simulink model "ARC_DTm"  (R2025b)
settings: Solver=FixedStepAuto  StartTime=0.0  StopTime=10080  FixedStep=1  RelTol=1e-3
PreLoadFcn:
  | %For Preload, set the working path
  | modelFolder = fileparts(which(bdroot));
  | addpath(genpath(modelFolder));
StartFcn:
  | tic
StopFcn:
  | fprintf("Sim Time: %.02f min", toc/60)
values from neighbouring files (symbols this model uses):
  batteryScenario = p.batteryScenario    [RUNSIM_ParameterSweep.m]    (also in _RUNSIM_ParameterSweep.m)
  Electricity_SalePriceModifier = 50/100    (= 0.5)    [RUNSIM_ParameterSweep.m]    (also in _RUNSIM_ParameterSweep.m)
  LUT = LUT_load.gamLUT    [RUNSIM_ParameterSweep.m]    (also in _RUNSIM_ParameterSweep.m)
  minimum_UF_system_flow = 5833    [RUNSIM_ParameterSweep.m]    (also in _RUNSIM_ParameterSweep.m)
  PROS1_recoveryrate = 61    [RUNSIM_ParameterSweep.m]    (also in _RUNSIM_ParameterSweep.m)
  PROS2_recoveryrate = 62    [RUNSIM_ParameterSweep.m]    (also in _RUNSIM_ParameterSweep.m)
  ROstabilization_time = p.ROstabilization_time    [RUNSIM_ParameterSweep.m]    (also in _RUNSIM_ParameterSweep.m)
  solarModifier = maximum_solar_generation / 300    [RUNSIM_ParameterSweep.m]    (also in _RUNSIM_ParameterSweep.m)
  TSRO_recoveryrate = 51    [RUNSIM_ParameterSweep.m]    (also in _RUNSIM_ParameterSweep.m)
  UF_RecoveryRate = 96    [RUNSIM_ParameterSweep.m]    (also in _RUNSIM_ParameterSweep.m)
undefined symbols (not defined in the file or in its folder): A_PROS1, A_PROS2, A_TSRO, B_PROS1, B_PROS2, B_TSRO, BW_Max_Time, BW_Max_Vol_gal, CEB_Max_Time, CEB_Max_Vol_gal, CIP_Max_Time, E, FF, h, L, w
libraries: simulink x40
(part 9 of 11)

== stateflow chart ARC_DTm/UF Maintenance Coordinator/arhive/UF_Operation State_6/UF6_Maintenance State ==
  settings: sampleTime=1  executeAtInitialization=1
  note: Unit State Machine — FIFO Maintenance Dispatch
      | This chart controls a single filtration unit through four operational states: Standby, Running, Await_Maintenance, BW_Maintenance, and CEB_Maintenance.
      | The unit begins in Standby, awaiting a startup command from the central dispatcher. Once commanded on, it enters Running, where it operates normally and tracks cumulative downtime. If a maintenance request is triggered, the unit transitions to Await_Maintenance, remaining online until the dispatcher confirms it can be released.
      | Two maintenance sequences are supported. A Backwash (BW) is a fixed-duration event (4 timesteps). A Chemically Enhanced Backwash (CEB) is a stochastic event lasting between 30 and 90 timesteps, sampled from a uniform distribution at entry. CEB is always followed by a BW cycle.
      | Upon completion of maintenance, the unit returns to Standby and re-enters the startup queue at the back, consistent with FIFO dispatching logic.
  note: Unit_cmd = 1 for running, 0 for off.
  state Standby
    during:
    %Unit is off, but awaiting startup.
    unit_in_startup_queue = 1;
    unit_in_operation = 0;
    %Ensure that the maintenance resets are occuring.
    maintenance_completion_indicator = 0;
  state Running
    entry:
    %Reset downtime timer
    cycle_downtime = 0;
    during:
    %Unit on, not in maint queue.
    unit_in_operation = 1;
    unit_in_maint_queue = 0;
  state Await_standby
    %Unit , Enter maint Queue
    during:
    unit_in_operation = 0;
    unit_in_maint_queue = 1;
  state Await_maintenance
    %Unit stays on, Enter maint Queue
    during:
    unit_in_operation = 1;
    unit_in_maint_queue = 1;
  state CEB_Maintenance
    %Unit is in chemically enhanced backwash. After CEB, do BW.
    %At start, determine a maintenance time within a uniform range of 30-60 min.
    entry:
    needed_maint_time = 30 + (60-30) * rand();
    %Exit state when time in maintenance is >= expected time.
    during:
    unit_in_operation = -1; %unit in maintenance
    %update maintenance time every step.
    cycle_downtime = cycle_downtime + 1;
  state BW_Maintenance
    entry:
    needed_maint_time = 1.5;
    %Exit state when time in maintenance is >= expected time.
    during:
    unit_in_operation = -1; %unit in maintenance
    %update maintenance time every step.
    cycle_downtime = cycle_downtime + 1;
    %ensure that the CEB is not continually reseting.
    maintenance_completion_indicator = 0;
  note: Maintenance Completion Indicator represents a signal to reset the counters at the UF unit tracking backwash cycles (signal = 2) and time in operations (signal = 1). These are pulse signals that reset integrators.
  (default) -> Running
  Standby -> Running : [startup_cmd == 1]{unit_in_startup_queue = 0;}
  Running -> (junction 44) [order 2] : [standby_cmd == 1]
  Running -> Await_maintenance [order 1] : [maint_req ~=0]
  (junction 22) -> Standby
  Await_standby -> (junction 47) : [standby_cmd == 1 && maint_cmd == 1]
  (junction 47) -> (junction 11)
  (junction 44) -> Await_standby
  Await_maintenance -> (junction 11) [order 2] : [maint_req == 1 && maint_cmd == 1] {unit_in_maint_queue = 0;}
  (junction 11) -> BW_Maintenance
  Await_maintenance -> CEB_Maintenance [order 1] : [maint_req == 2 && maint_cmd ==1]
  CEB_Maintenance -> BW_Maintenance : [after(needed_maint_time, tick)]{maintenance_completion_indicator = 2;}
  BW_Maintenance -> (junction 22) : [after(needed_maint_time, tick)]
      | {maintenance_completion_indicator = 1;}
  data: maint_cmd input; maint_req input; standby_cmd input; startup_cmd input; unit_in_maint_queue output; unit_in_startup_queue output; cycle_downtime local; needed_maint_time local; unit_in_operation output; maintenance_completion_indicator output

== matlab function ARC_DTm/Plant Setpoints/Number PRO S1 Units ==
  data: flows output; max_flow_per_unit input; flow_actual input; Number_in_service output; flow_setpoint input; prev_flows input; Stabilization_Time input; ROstabilization_time input
function [flows, Number_in_service] = ROUnits(max_flow_per_unit, flow_actual, flow_setpoint, prev_flows, Stabilization_Time,ROstabilization_time)

flows = zeros( 4,1);
demanded_flows = zeros(4,1);

current_units = sum(prev_flows>0);
target_units = min(ceil(flow_setpoint / max_flow_per_unit), 4);
% Unit count driven by setpoint
if Stabilization_Time >= ROstabilization_time

    %during rampdown, avoid shutting off all units immediately
    if flow_setpoint == 0 && flow_actual ~= 0
        Number_in_service = max(target_units, current_units);
    else
        Number_in_service = target_units;
    end
else
    Number_in_service = 1;
end

% Target each unit is heading toward (based on setpoint)
demanded_flows(1:Number_in_service) = flow_setpoint / Number_in_service;

% Change in total actual flow this timestep (this should be throttled by
% rate limiter) on flow_actual.
delta_Q_total = flow_actual - sum(prev_flows); %total change in flow this timestep
avg_delta_Q_unit = delta_Q_total/Number_in_service; %benchmark to limit rate change.

% Distribute that delta evenly across active units, move toward demanded
delta_Q_unit_demanded = zeros(4,1); %demanded change in flows to reach setpoint
delta_Q = zeros(4,1); %actual change in flows this step.
for i = 1:4

        %get demanded change in flows.
        delta_Q_unit_demanded(i) = demanded_flows(i) - prev_flows(i);  
         
        delta_Q(i) = sign(delta_Q_unit_demanded(i)) * min(abs(delta_Q_unit_demanded(i)), abs(delta_Q_total/Number_in_service));


        flows(i) = prev_flows(i) + delta_Q(i);
        

        delta_Q_total = delta_Q_total - delta_Q(i);
end

end

== stateflow chart ARC_DTm/UF Maintenance Coordinator/arhive/UF_Operation State_7/UF7_Maintenance State ==
  settings: sampleTime=1  executeAtInitialization=1
  note: Unit State Machine — FIFO Maintenance Dispatch
      | This chart controls a single filtration unit through four operational states: Standby, Running, Await_Maintenance, BW_Maintenance, and CEB_Maintenance.
      | The unit begins in Standby, awaiting a startup command from the central dispatcher. Once commanded on, it enters Running, where it operates normally and tracks cumulative downtime. If a maintenance request is triggered, the unit transitions to Await_Maintenance, remaining online until the dispatcher confirms it can be released.
      | Two maintenance sequences are supported. A Backwash (BW) is a fixed-duration event (4 timesteps). A Chemically Enhanced Backwash (CEB) is a stochastic event lasting between 30 and 90 timesteps, sampled from a uniform distribution at entry. CEB is always followed by a BW cycle.
      | Upon completion of maintenance, the unit returns to Standby and re-enters the startup queue at the back, consistent with FIFO dispatching logic.
  note: Unit_cmd = 1 for running, 0 for off.
  state Standby
    during:
    %Unit is off, but awaiting startup.
    unit_in_startup_queue = 1;
    unit_in_operation = 0;
    %Ensure that the maintenance resets are occuring.
    maintenance_completion_indicator = 0;
  state Running
    entry:
    %Reset downtime timer
    cycle_downtime = 0;
    during:
    %Unit on, not in maint queue.
    unit_in_operation = 1;
    unit_in_maint_queue = 0;
  state Await_standby
    %Unit , Enter maint Queue
    during:
    unit_in_operation = 0;
    unit_in_maint_queue = 1;
  state Await_maintenance
    %Unit stays on, Enter maint Queue
    during:
    unit_in_operation = 1;
    unit_in_maint_queue = 1;
  state CEB_Maintenance
    %Unit is in chemically enhanced backwash. After CEB, do BW.
    %At start, determine a maintenance time within a uniform range of 30-60 min.
    entry:
    needed_maint_time = 30 + (60-30) * rand();
    %Exit state when time in maintenance is >= expected time.
    during:
    unit_in_operation = -1; %unit in maintenance
    %update maintenance time every step.
    cycle_downtime = cycle_downtime + 1;
  state BW_Maintenance
    entry:
    needed_maint_time = 1.5;
    %Exit state when time in maintenance is >= expected time.
    during:
    unit_in_operation = -1; %unit in maintenance
    %update maintenance time every step.
    cycle_downtime = cycle_downtime + 1;
    %ensure that the CEB is not continually reseting.
    maintenance_completion_indicator = 0;
  note: Maintenance Completion Indicator represents a signal to reset the counters at the UF unit tracking backwash cycles (signal = 2) and time in operations (signal = 1). These are pulse signals that reset integrators.
  (default) -> Running
  Standby -> Running : [startup_cmd == 1]{unit_in_startup_queue = 0;}
  Running -> (junction 44) [order 2] : [standby_cmd == 1]
  Running -> Await_maintenance [order 1] : [maint_req ~=0]
  (junction 22) -> Standby
  Await_standby -> (junction 47) : [standby_cmd == 1 && maint_cmd == 1]
  (junction 47) -> (junction 11)
  (junction 44) -> Await_standby
  Await_maintenance -> (junction 11) [order 2] : [maint_req == 1 && maint_cmd == 1] {unit_in_maint_queue = 0;}
  (junction 11) -> BW_Maintenance
  Await_maintenance -> CEB_Maintenance [order 1] : [maint_req == 2 && maint_cmd ==1]
  CEB_Maintenance -> BW_Maintenance : [after(needed_maint_time, tick)]{maintenance_completion_indicator = 2;}
  BW_Maintenance -> (junction 22) : [after(needed_maint_time, tick)]
      | {maintenance_completion_indicator = 1;}
  data: maint_cmd input; maint_req input; standby_cmd input; startup_cmd input; unit_in_maint_queue output; unit_in_startup_queue output; cycle_downtime local; needed_maint_time local; unit_in_operation output; maintenance_completion_indicator output

== stateflow chart ARC_DTm/UF Maintenance Coordinator/arhive/UF_Operation State_8/UF8_Maintenance State ==
  settings: sampleTime=1  executeAtInitialization=1
  note: Unit State Machine — FIFO Maintenance Dispatch
      | This chart controls a single filtration unit through four operational states: Standby, Running, Await_Maintenance, BW_Maintenance, and CEB_Maintenance.
      | The unit begins in Standby, awaiting a startup command from the central dispatcher. Once commanded on, it enters Running, where it operates normally and tracks cumulative downtime. If a maintenance request is triggered, the unit transitions to Await_Maintenance, remaining online until the dispatcher confirms it can be released.
      | Two maintenance sequences are supported. A Backwash (BW) is a fixed-duration event (4 timesteps). A Chemically Enhanced Backwash (CEB) is a stochastic event lasting between 30 and 90 timesteps, sampled from a uniform distribution at entry. CEB is always followed by a BW cycle.
      | Upon completion of maintenance, the unit returns to Standby and re-enters the startup queue at the back, consistent with FIFO dispatching logic.
  note: Unit_cmd = 1 for running, 0 for off.
  state Standby
    during:
    %Unit is off, but awaiting startup.
    unit_in_startup_queue = 1;
    unit_in_operation = 0;
    %Ensure that the maintenance resets are occuring.
    maintenance_completion_indicator = 0;
  state Running
    entry:
    %Reset downtime timer
    cycle_downtime = 0;
    during:
    %Unit on, not in maint queue.
    unit_in_operation = 1;
    unit_in_maint_queue = 0;
  state Await_standby
    %Unit , Enter maint Queue
    during:
    unit_in_operation = 0;
    unit_in_maint_queue = 1;
  state Await_maintenance
    %Unit stays on, Enter maint Queue
    during:
    unit_in_operation = 1;
    unit_in_maint_queue = 1;
  state CEB_Maintenance
    %Unit is in chemically enhanced backwash. After CEB, do BW.
    %At start, determine a maintenance time within a uniform range of 30-60 min.
    entry:
    needed_maint_time = 30 + (60-30) * rand();
    %Exit state when time in maintenance is >= expected time.
    during:
    unit_in_operation = -1; %unit in maintenance
    %update maintenance time every step.
    cycle_downtime = cycle_downtime + 1;
  state BW_Maintenance
    entry:
    needed_maint_time = 1.5;
    %Exit state when time in maintenance is >= expected time.
    during:
    unit_in_operation = -1; %unit in maintenance
    %update maintenance time every step.
    cycle_downtime = cycle_downtime + 1;
    %ensure that the CEB is not continually reseting.
    maintenance_completion_indicator = 0;
  note: Maintenance Completion Indicator represents a signal to reset the counters at the UF unit tracking backwash cycles (signal = 2) and time in operations (signal = 1). These are pulse signals that reset integrators.
  (default) -> Running
  Standby -> Running : [startup_cmd == 1]{unit_in_startup_queue = 0;}
  Running -> (junction 44) [order 2] : [standby_cmd == 1]
  Running -> Await_maintenance [order 1] : [maint_req ~=0]
  (junction 22) -> Standby
  Await_standby -> (junction 47) : [standby_cmd == 1 && maint_cmd == 1]
  (junction 47) -> (junction 11)
  (junction 44) -> Await_standby
  Await_maintenance -> (junction 11) [order 2] : [maint_req == 1 && maint_cmd == 1] {unit_in_maint_queue = 0;}
  (junction 11) -> BW_Maintenance
  Await_maintenance -> CEB_Maintenance [order 1] : [maint_req == 2 && maint_cmd ==1]
  CEB_Maintenance -> BW_Maintenance : [after(needed_maint_time, tick)]{maintenance_completion_indicator = 2;}
  BW_Maintenance -> (junction 22) : [after(needed_maint_time, tick)]
      | {maintenance_completion_indicator = 1;}
  data: maint_cmd input; maint_req input; standby_cmd input; startup_cmd input; unit_in_maint_queue output; unit_in_startup_queue output; cycle_downtime local; needed_maint_time local; unit_in_operation output; maintenance_completion_indicator output

== stateflow chart ARC_DTm/UF Maintenance Coordinator/arhive/UF_Operation State_9/UF9_Maintenance State ==
  settings: sampleTime=1  executeAtInitialization=1
  note: Unit State Machine — FIFO Maintenance Dispatch
      | This chart controls a single filtration unit through four operational states: Standby, Running, Await_Maintenance, BW_Maintenance, and CEB_Maintenance.
      | The unit begins in Standby, awaiting a startup command from the central dispatcher. Once commanded on, it enters Running, where it operates normally and tracks cumulative downtime. If a maintenance request is triggered, the unit transitions to Await_Maintenance, remaining online until the dispatcher confirms it can be released.
      | Two maintenance sequences are supported. A Backwash (BW) is a fixed-duration event (4 timesteps). A Chemically Enhanced Backwash (CEB) is a stochastic event lasting between 30 and 90 timesteps, sampled from a uniform distribution at entry. CEB is always followed by a BW cycle.
      | Upon completion of maintenance, the unit returns to Standby and re-enters the startup queue at the back, consistent with FIFO dispatching logic.
  note: Unit_cmd = 1 for running, 0 for off.
  state Standby
    during:
    %Unit is off, but awaiting startup.
    unit_in_startup_queue = 1;
    unit_in_operation = 0;
    %Ensure that the maintenance resets are occuring.
    maintenance_completion_indicator = 0;
  state Running
    entry:
    %Reset downtime timer
    cycle_downtime = 0;
    during:
    %Unit on, not in maint queue.
    unit_in_operation = 1;
    unit_in_maint_queue = 0;
  state Await_standby
    %Unit , Enter maint Queue
    during:
    unit_in_operation = 0;
    unit_in_maint_queue = 1;
  state Await_maintenance
    %Unit stays on, Enter maint Queue
    during:
    unit_in_operation = 1;
    unit_in_maint_queue = 1;
  state CEB_Maintenance
    %Unit is in chemically enhanced backwash. After CEB, do BW.
    %At start, determine a maintenance time within a uniform range of 30-60 min.
    entry:
    needed_maint_time = 30 + (60-30) * rand();
    %Exit state when time in maintenance is >= expected time.
    during:
    unit_in_operation = -1; %unit in maintenance
    %update maintenance time every step.
    cycle_downtime = cycle_downtime + 1;
  state BW_Maintenance
    entry:
    needed_maint_time = 1.5;
    %Exit state when time in maintenance is >= expected time.
    during:
    unit_in_operation = -1; %unit in maintenance
    %update maintenance time every step.
    cycle_downtime = cycle_downtime + 1;
    %ensure that the CEB is not continually reseting.
    maintenance_completion_indicator = 0;
  note: Maintenance Completion Indicator represents a signal to reset the counters at the UF unit tracking backwash cycles (signal = 2) and time in operations (signal = 1). These are pulse signals that reset integrators.
  (default) -> Running
  Standby -> Running : [startup_cmd == 1]{unit_in_startup_queue = 0;}
  Running -> (junction 44) [order 2] : [standby_cmd == 1]
  Running -> Await_maintenance [order 1] : [maint_req ~=0]
  (junction 22) -> Standby
  Await_standby -> (junction 47) : [standby_cmd == 1 && maint_cmd == 1]
  (junction 47) -> (junction 11)
  (junction 44) -> Await_standby
  Await_maintenance -> (junction 11) [order 2] : [maint_req == 1 && maint_cmd == 1] {unit_in_maint_queue = 0;}
  (junction 11) -> BW_Maintenance
  Await_maintenance -> CEB_Maintenance [order 1] : [maint_req == 2 && maint_cmd ==1]
  CEB_Maintenance -> BW_Maintenance : [after(needed_maint_time, tick)]{maintenance_completion_indicator = 2;}
  BW_Maintenance -> (junction 22) : [after(needed_maint_time, tick)]
      | {maintenance_completion_indicator = 1;}
  data: maint_cmd input; maint_req input; standby_cmd input; startup_cmd input; unit_in_maint_queue output; unit_in_startup_queue output; cycle_downtime local; needed_maint_time local; unit_in_operation output; maintenance_completion_indicator output

== matlab function ARC_DTm/Plant Setpoints/Number UF Units ==
  data: flows output; max_flow_per_unit input; flow_actual input; Number_in_service output; flow_setpoint input; prev_flows input
function [flows, Number_in_service] = UFUnits(max_flow_per_unit, flow_actual, flow_setpoint, prev_flows)

num_units_available = 10; 
flows = zeros( num_units_available,1);
demanded_flows = zeros(num_units_available,1);

current_units = sum(prev_flows>0);
target_units = min(ceil(flow_setpoint / max_flow_per_unit), num_units_available);
% Unit count driven by setpoint

    %during rampdown, avoid shutting off all units immediately
    if flow_setpoint == 0 && flow_actual ~= 0
        Number_in_service = max(target_units, current_units);
    else
        Number_in_service = target_units;
    end

% Target each unit is heading toward (based on setpoint)
demanded_flows(1:Number_in_service) = flow_setpoint / Number_in_service;

% Change in total actual flow this timestep (this should be throttled by
% rate limiter) on flow_actual.
delta_Q_total = flow_actual - sum(prev_flows); %total change in flow this timestep
avg_delta_Q_unit = delta_Q_total/Number_in_service; %benchmark to limit rate change.

% Distribute that delta evenly across active units, move toward demanded
delta_Q_unit_demanded = zeros(num_units_available,1); %demanded change in flows to reach setpoint
delta_Q = zeros(num_units_available,1); %actual change in flows this step.
for i = 1:num_units_available

        %get demanded change in flows.
        delta_Q_unit_demanded(i) = demanded_flows(i) - prev_flows(i);  
         
        delta_Q(i) = sign(delta_Q_unit_demanded(i)) * min(abs(delta_Q_unit_demanded(i)), abs(delta_Q_total/Number_in_service));


        flows(i) = prev_flows(i) + delta_Q(i);
        

        delta_Q_total = delta_Q_total - delta_Q(i);
end

end

== matlab function ARC_DTm/UF_Feed_Manifold/MATLAB Function ==
  data: UF_FeedPressure_vector output; prescribed_feedflow_vec input; UFPump_Pressure_Setpoint output; membrane_conductance_vec input; UF_PermeatePressure_vec input; dP_valve_req output
function [UF_FeedPressure_vector, UFPump_Pressure_Setpoint, dP_valve_req] = UF_ControlValves(prescribed_feedflow_vec, membrane_conductance_vec, UF_PermeatePressure_vec)

%initialize vectors
N = length(membrane_conductance_vec);

UF_FeedPressure_vector = zeros(N,1);
dP_valve_req = zeros(N,1);

%-------------------------------------------
%---- Step 1: Get desired permeate flows----
%-------------------------------------------

UFrecovery = .96; %constant 96% recovery
prescribed_permflow_vec = prescribed_feedflow_vec * UFrecovery;

%--------------------------------------------------------
%---- Step 2: Get feedpressure demanded for each unit----
%--------------------------------------------------------

% Required feed pressure for each active skid
for i = 1:N
    if prescribed_permflow_vec(i) >0
        UF_FeedPressure_vector(i) = prescribed_permflow_vec(i) / membrane_conductance_vec(i) + UF_PermeatePressure_vec(i);
    else
        UF_FeedPressure_vector(i) = 0;
    end

end

%--------------------------------------------------------
%---- Step 3: Get feedpressure demanded fropm pumps------
%--------------------------------------------------------

% Pump pressure setpoint
UFPump_Pressure_Setpoint = max(UF_FeedPressure_vector);



%--------------------------------------------------------
%---- Step 4: Get valve pressure drop -------------------
%--------------------------------------------------------
% Required valve pressure drop, not needed, but can be good to plot.
for i = 1:N
    if prescribed_permflow_vec(i) >0
        dP_valve_req(i) = UFPump_Pressure_Setpoint - UF_FeedPressure_vector(i);
        
    %if unit off, close valve
    else
        dP_valve_req(i) = 0;
    end


end

== matlab function ARC_DTm/RO Permeate Manifold/MATLAB Function ==
  data: max_flow_per_unit input; UVflows output; min_flow_per_unit input; flow_setpoint input; Number_in_service output
function [UVflows, Number_in_service] = UVAOPUnits(max_flow_per_unit, min_flow_per_unit, flow_setpoint)
% Pre-allocate outputs
UVflows = zeros(2, 1);

% --- Below minimum: no units run ---
if flow_setpoint < min_flow_per_unit
    Number_in_service = 0;
    return
end

% --- One unit can handle it: max out unit 1, unit 2 gets remainder ---
if flow_setpoint <= max_flow_per_unit
    Number_in_service = 1;
    UVflows(1) = flow_setpoint;
    return
end

% --- Flow exceeds one unit max: fill unit 1, give remainder to unit 2 ---
remainder = flow_setpoint - max_flow_per_unit;

if remainder >= min_flow_per_unit
    % Remainder is enough to run unit 2 — max out unit 1
    Number_in_service = 2;
    UVflows(1) = max_flow_per_unit;
    UVflows(2) = remainder;
else
    % Remainder too low for unit 2 — split evenly instead
    Number_in_service = 2;
    UVflows(1) = flow_setpoint / 2;
    UVflows(2) = flow_setpoint / 2;
end

end

== matlab function ARC_DTm/UF Pumping/MATLAB Function ==
  data: max_flow_per_unit input; min_flow_per_unit input; flow_setpoint input; flow_actual input; prev_flows input; speeds output; h_des input; powers output; effs output; flows output; totalPower output; full_flow_units output
function [speeds, powers, effs, flows, totalPower, full_flow_units] = Pumps_in_parallel_maximize(max_flow_per_unit, min_flow_per_unit, flow_setpoint, flow_actual, prev_flows,h_des)

persistent pump_data
if isempty(pump_data)
    loaded = coder.load('Pumps\LookupTables.mat');
    pump_data = loaded.pump.UF_pump;
end

num_units_available =4;

% Pre-allocate outputs
speeds = zeros(num_units_available,1);
powers = zeros(num_units_available,1);
effs   = zeros(num_units_available,1);
flow_sp  = zeros(num_units_available,1);
flows  = zeros(num_units_available,1);

%Primary Units split flow evenly.
%Round down number of units in service that are maxed out
full_flow_units = min(floor(flow_setpoint / max_flow_per_unit), num_units_available - 1);

%ensure that support_flow_setpoint is above minimum value for pump
support_flow = rem(flow_setpoint, max_flow_per_unit);
if support_flow < min_flow_per_unit
    support_flow_sp = min_flow_per_unit;
    flow_SP_per_maxed_unit = (flow_setpoint - support_flow_sp)/full_flow_units;
    Number_in_service = full_flow_units+1;

elseif support_flow == 0
    Number_in_service = full_flow_units;
    support_flow_sp = support_flow;
    flow_SP_per_maxed_unit = max_flow_per_unit;
else 
    support_flow_sp = support_flow;
    flow_SP_per_maxed_unit = max_flow_per_unit;
    Number_in_service = full_flow_units+1;

end



%Assign flow setpoints for adaptive distribution during ramping periods
flow_sp(1:full_flow_units) = flow_SP_per_maxed_unit;
flow_sp(Number_in_service) = support_flow_sp;

% Distribute that delta evenly across active units, move toward demanded
delta_Q_unit_demanded =  zeros(1,num_units_available); %demanded change in flows to reach setpoint
delta_Q =  zeros(1,num_units_available); %actual change in flows this step.
delta_Q_total = flow_actual - sum(prev_flows); %total change in flow this timestep

units_left = Number_in_service;
%allocate flow to units in service 
for i = 1:Number_in_service

        %get demanded change in flows.
        delta_Q_unit_demanded(i) = flow_sp(i) - prev_flows(i);  
        
        %ramp up should be split between each unit
        %if it can reach its goal, do so. Otherwise, follow the total
        %actual change in flow per unit
        delta_Q(i) = sign(delta_Q_unit_demanded(i)) * min(abs(delta_Q_unit_demanded(i)), abs(delta_Q_total/units_left)); 

        flows(i) = prev_flows(i) + delta_Q(i);


        delta_Q_total = delta_Q_total - delta_Q(i);
        units_left = units_left - 1;
end


for i = 1:num_units_available

    Q_des = flows(i);

    if Q_des > 0

        speed = interp2(pump_data.Q_grid, pump_data.H_grid, ...
            pump_data.speed_grid, Q_des, h_des, 'linear');

        if ~isnan(speed)
            power = interp2(pump_data.H_grid_pwr, pump_data.S_grid_pwr, ...
                pump_data.power_grid, h_des, speed, 'linear');

            eff = interp2(pump_data.H_grid_pwr, pump_data.S_grid_pwr, ...
                pump_data.total_eff_grid, h_des, speed, 'linear');
        else
            power = NaN;
            eff = NaN;
        end

        % Fallback only for low-end conditions
        if isnan(speed) || isnan(power)

            Q_min = min(pump_data.Q_grid(:));
            h_min = min(pump_data.H_grid(:));

            speed_min = interp2(pump_data.Q_grid, pump_data.H_grid, ...
                pump_data.speed_grid, Q_min, h_min, 'linear');

            P_min = interp2(pump_data.H_grid_pwr, pump_data.S_grid_pwr, ...
                pump_data.power_grid, h_min, speed_min, 'linear');

            if Q_des < Q_min
                speed = speed_min / Q_min * Q_des;
                power = (speed / speed_min)^3 * P_min;

            elseif h_des < h_min
                speed = speed_min * (h_des / h_min)^(1/2);
                power = (speed / speed_min)^3 * P_min;

            else
                speed = 0;
                power = 0;
            end

            eff = NaN;
        end

        speeds(i) = speed;
        powers(i) = power;
        effs(i) = eff;

    end
end
    totalPower = sum(powers);
end

== matlab function ARC_DTm/PROS1_1/MATLAB Function1 ==
  data: W input; h input; dh output
function dh = hydDiameter(W,h)

dh = 2*h*W/(h+W);

== matlab function ARC_DTm/PROS1_1/MATLAB Function2 ==
  data: cperm input; cbrine output; Qperm input; Qbrine input; Qfeed input; cfeed input
function cbrine = fcn(cperm, Qperm, Qbrine, Qfeed, cfeed)

Wtot = Qfeed * cfeed;
Wperm = cperm * Qperm;

%account for NaN
if Qbrine > 0
cbrine = (Wtot - Wperm)/Qbrine;
else
    cbrine = 0;
end

== matlab function ARC_DTm/PROS1_1/Subsystem/MATLAB Function ==
  data: T input; Pfeed input; Pperm input; A input; B input; cfeed input; cperm_prev input; Jw_prev input; dh input; L input; u input; Jw output; cperm output; deltaPi_bar output
function [Jw, cperm, deltaPi_bar] = ROBehavior(T, Pfeed, Pperm, A, B, cfeed, cperm_prev,Jw_prev, dh, L, u)
    
    cmem = ConP(cfeed, T, dh, L, u, Jw_prev);

    [pi_feed] = osmPres(T,cmem);
    [pi_perm] = osmPres(T,cperm_prev);
    
    deltaPi_bar = pi_feed - pi_perm;
    [Jw, cperm] = solutionDiffusion(T, Pfeed, Pperm, A, B, cmem, cperm_prev, pi_feed, pi_perm);
   
end

== matlab function ARC_DTm/PROS1_3_Pump/MATLAB Function ==
  data: Q_des input; speed output; h_des input; power output
function [speed, power] = query_pump(Q_des, h_des)
% QUERY_PUMP Find pump speed, power, and efficiency given flow and head
%MUST UPDATE the pump_data call
%
% Inputs:
%   Q_des     - Desired flow rate (gpm)
%   h_des     - Desired added head (ft)
%   pump_data - Struct for a single pump (e.g. pump.pump_A)
%
% Outputs:
%   speed      - Interpolated speed
%   power      - Interpolated power
%   total_eff  - Interpolated total efficiency (%)
%   totalPower - Power demand accounting for efficiency (power / total_eff / 100)

persistent pump_data Q_min h_min speed_min  P_min
if isempty(pump_data)
    loaded = coder.load('Pumps\LookupTables.mat');
    pump_data = loaded.pump.RO_feed_pump;
    Q_min = min(pump_data.Q_grid(:));
    h_min = min(pump_data.H_grid(:));

    speed_min = interp2(pump_data.Q_grid, pump_data.H_grid, pump_data.speed_grid, Q_min, h_min, 'linear');
    P_min = interp2(pump_data.H_grid_pwr, pump_data.S_grid_pwr, pump_data.power_grid, h_min, speed_min, 'linear');

end

%zero flow conditions not present in the existing dataset.
if Q_des <= .1 * Q_min
    speed = 0;
    power = 0;
    total_eff = 0;
    return
end

% Normal lookup
speed = interp2(pump_data.Q_grid, pump_data.H_grid, ...
    pump_data.speed_grid, Q_des, h_des, 'linear');

if ~isnan(speed)
    power = interp2(pump_data.H_grid_pwr, pump_data.S_grid_pwr, ...
        pump_data.power_grid, h_des, speed, 'linear');
else
    power = NaN;
end

% Fallback only for low-end conditions
if isnan(speed) || isnan(power)
    if Q_des < Q_min       
        speed = speed_min / Q_min * Q_des;
         power = (speed / speed_min)^3 * P_min;

    else if h_des < h_min
        speed = speed_min * (h_des / h_min)^(1/2);
        power = (speed / speed_min)^3 * P_min;

    else
        speed = 0;
        power = 0;
    end


end

end

== matlab function ARC_DTm/PROS1_3/MATLAB Function1 ==
  data: W input; h input; dh output
function dh = hydDiameter(W,h)

dh = 2*h*W/(h+W);

== matlab function ARC_DTm/PROS1_1_Pump/MATLAB Function ==
  data: Q_des input; speed output; h_des input; power output
function [speed, power] = query_pump(Q_des, h_des)
% QUERY_PUMP Find pump speed, power, and efficiency given flow and head
%MUST UPDATE the pump_data call
%
% Inputs:
%   Q_des     - Desired flow rate (gpm)
%   h_des     - Desired added head (ft)
%   pump_data - Struct for a single pump (e.g. pump.pump_A)
%
% Outputs:
%   speed      - Interpolated speed
%   power      - Interpolated power
%   total_eff  - Interpolated total efficiency (%)
%   totalPower - Power demand accounting for efficiency (power / total_eff / 100)

persistent pump_data Q_min h_min speed_min  P_min
if isempty(pump_data)
    loaded = coder.load('Pumps\LookupTables.mat');
    pump_data = loaded.pump.RO_feed_pump;
    Q_min = min(pump_data.Q_grid(:));
    h_min = min(pump_data.H_grid(:));

    speed_min = interp2(pump_data.Q_grid, pump_data.H_grid, pump_data.speed_grid, Q_min, h_min, 'linear');
    P_min = interp2(pump_data.H_grid_pwr, pump_data.S_grid_pwr, pump_data.power_grid, h_min, speed_min, 'linear');

end

%zero flow conditions not present in the existing dataset.
if Q_des <= .1 * Q_min
    speed = 0;
    power = 0;
    total_eff = 0;
    return
end

% Normal lookup
speed = interp2(pump_data.Q_grid, pump_data.H_grid, ...
    pump_data.speed_grid, Q_des, h_des, 'linear');

if ~isnan(speed)
    power = interp2(pump_data.H_grid_pwr, pump_data.S_grid_pwr, ...
        pump_data.power_grid, h_des, speed, 'linear');
else
    power = NaN;
end

% Fallback only for low-end conditions
if isnan(speed) || isnan(power)
    if Q_des < Q_min       
        speed = speed_min / Q_min * Q_des;
         power = (speed / speed_min)^3 * P_min;

    else if h_des < h_min
        speed = speed_min * (h_des / h_min)^(1/2);
        power = (speed / speed_min)^3 * P_min;

    else
        speed = 0;
        power = 0;
    end


end

end

== matlab function ARC_DTm/PROS2_2_Pump/MATLAB Function1 ==
  data: Q_des input; speed output; h_des input; power output
function [speed, power] = query_pump(Q_des, h_des)
% QUERY_PUMP Find pump speed, power, and efficiency given flow and head
%MUST UPDATE the pump_data call
%
% Inputs:
%   Q_des     - Desired flow rate (gpm)
%   h_des     - Desired added head (ft)
%   pump_data - Struct for a single pump (e.g. pump.pump_A)
%
% Outputs:
%   speed      - Interpolated speed
%   power      - Interpolated power
%   total_eff  - Interpolated total efficiency (%)
%   totalPower - Power demand accounting for efficiency (power / total_eff / 100)

persistent pump_data Q_min h_min speed_min  P_min
if isempty(pump_data)
    loaded = coder.load('Pumps\LookupTables.mat');
    pump_data = loaded.pump.RO_IS_pump;
    Q_min = min(pump_data.Q_grid(:));
    h_min = min(pump_data.H_grid(:));

    speed_min = interp2(pump_data.Q_grid, pump_data.H_grid, pump_data.speed_grid, Q_min, h_min, 'linear');
    P_min = interp2(pump_data.H_grid_pwr, pump_data.S_grid_pwr, pump_data.power_grid, h_min, speed_min, 'linear');

end

%zero flow conditions not present in the existing dataset.
if Q_des <= .1 * Q_min
    speed = 0;
    power = 0;
    total_eff = 0;
    return
end

% Normal lookup
speed = interp2(pump_data.Q_grid, pump_data.H_grid, ...
    pump_data.speed_grid, Q_des, h_des, 'linear');

if ~isnan(speed)
    power = interp2(pump_data.H_grid_pwr, pump_data.S_grid_pwr, ...
        pump_data.power_grid, h_des, speed, 'linear');
else
    power = NaN;
end

% Fallback only for low-end conditions
if isnan(speed) || isnan(power)
    if Q_des < Q_min       
        speed = speed_min / Q_min * Q_des;
         power = (speed / speed_min)^3 * P_min;

    else if h_des < h_min
        speed = speed_min * (h_des / h_min)^(1/2);
        power = (speed / speed_min)^3 * P_min;

    else
        speed = 0;
        power = 0;
    end


end


end

== matlab function ARC_DTm/PROS2_1/MATLAB Function1 ==
  data: W input; h input; dh output
function dh = hydDiameter(W,h)

dh = 2*h*W/(h+W);

== matlab function ARC_DTm/PROS2_1/MATLAB Function2 ==
  data: cperm input; cbrine output; Qperm input; Qbrine input; Qfeed input; cfeed input
function cbrine = fcn(cperm, Qperm, Qbrine, Qfeed, cfeed)

Wtot = Qfeed * cfeed;
Wperm = cperm * Qperm;

%account for NaN
if Qbrine > 0
cbrine = (Wtot - Wperm)/Qbrine;
else
    cbrine = 0;
end

== matlab function ARC_DTm/PROS2_1/Subsystem/MATLAB Function ==
  data: T input; Pfeed input; Pperm input; A input; B input; cfeed input; cperm_prev input; Jw_prev input; dh input; L input; u input; Jw output; cperm output; deltaPi_bar output
function [Jw, cperm, deltaPi_bar] = ROBehavior(T, Pfeed, Pperm, A, B, cfeed, cperm_prev,Jw_prev, dh, L, u)
   
    cmem = ConP(cfeed, T, dh, L, u, Jw_prev);
    [pi_feed] = osmPres(T,cmem);
    [pi_perm] = osmPres(T,cperm_prev);
    
    deltaPi_bar = pi_feed - pi_perm;
    [Jw, cperm] = solutionDiffusion(T, Pfeed, Pperm, A, B, cmem, cperm_prev, pi_feed, pi_perm);
end

== matlab function ARC_DTm/PROS1_4_Pump/MATLAB Function ==
  data: Q_des input; speed output; h_des input; power output
function [speed, power] = query_pump(Q_des, h_des)
% QUERY_PUMP Find pump speed, power, and efficiency given flow and head
%MUST UPDATE the pump_data call
%
% Inputs:
%   Q_des     - Desired flow rate (gpm)
%   h_des     - Desired added head (ft)
%   pump_data - Struct for a single pump (e.g. pump.pump_A)
%
% Outputs:
%   speed      - Interpolated speed
%   power      - Interpolated power
%   total_eff  - Interpolated total efficiency (%)
%   totalPower - Power demand accounting for efficiency (power / total_eff / 100)

persistent pump_data Q_min h_min speed_min  P_min
if isempty(pump_data)
    loaded = coder.load('Pumps\LookupTables.mat');
    pump_data = loaded.pump.RO_feed_pump;
    Q_min = min(pump_data.Q_grid(:));
    h_min = min(pump_data.H_grid(:));

    speed_min = interp2(pump_data.Q_grid, pump_data.H_grid, pump_data.speed_grid, Q_min, h_min, 'linear');
    P_min = interp2(pump_data.H_grid_pwr, pump_data.S_grid_pwr, pump_data.power_grid, h_min, speed_min, 'linear');

end

%zero flow conditions not present in the existing dataset.
if Q_des <= .1 * Q_min
    speed = 0;
    power = 0;
    total_eff = 0;
    return
end

% Normal lookup
speed = interp2(pump_data.Q_grid, pump_data.H_grid, ...
    pump_data.speed_grid, Q_des, h_des, 'linear');

if ~isnan(speed)
    power = interp2(pump_data.H_grid_pwr, pump_data.S_grid_pwr, ...
        pump_data.power_grid, h_des, speed, 'linear');
else
    power = NaN;
end

% Fallback only for low-end conditions
if isnan(speed) || isnan(power)
    if Q_des < Q_min       
        speed = speed_min / Q_min * Q_des;
         power = (speed / speed_min)^3 * P_min;

    else if h_des < h_min
        speed = speed_min * (h_des / h_min)^(1/2);
        power = (speed / speed_min)^3 * P_min;

    else
        speed = 0;
        power = 0;
    end


end

end

== matlab function ARC_DTm/PROS1_4/MATLAB Function1 ==
  data: W input; h input; dh output
function dh = hydDiameter(W,h)

dh = 2*h*W/(h+W);

== matlab function ARC_DTm/PROS1_2_Pump/MATLAB Function ==
  data: Q_des input; speed output; h_des input; power output
function [speed, power] = query_pump(Q_des, h_des)
% QUERY_PUMP Find pump speed, power, and efficiency given flow and head
%MUST UPDATE the pump_data call
%
% Inputs:
%   Q_des     - Desired flow rate (gpm)
%   h_des     - Desired added head (ft)
%   pump_data - Struct for a single pump (e.g. pump.pump_A)
%
% Outputs:
%   speed      - Interpolated speed
%   power      - Interpolated power
%   total_eff  - Interpolated total efficiency (%)
%   totalPower - Power demand accounting for efficiency (power / total_eff / 100)

persistent pump_data Q_min h_min speed_min  P_min
if isempty(pump_data)
    loaded = coder.load('Pumps\LookupTables.mat');
    pump_data = loaded.pump.RO_feed_pump;
    Q_min = min(pump_data.Q_grid(:));
    h_min = min(pump_data.H_grid(:));

    speed_min = interp2(pump_data.Q_grid, pump_data.H_grid, pump_data.speed_grid, Q_min, h_min, 'linear');
    P_min = interp2(pump_data.H_grid_pwr, pump_data.S_grid_pwr, pump_data.power_grid, h_min, speed_min, 'linear');

end

%zero flow conditions not present in the existing dataset.
if Q_des <= .1 * Q_min
    speed = 0;
    power = 0;
    total_eff = 0;
    return
end

% Normal lookup
speed = interp2(pump_data.Q_grid, pump_data.H_grid, ...
    pump_data.speed_grid, Q_des, h_des, 'linear');

if ~isnan(speed)
    power = interp2(pump_data.H_grid_pwr, pump_data.S_grid_pwr, ...
        pump_data.power_grid, h_des, speed, 'linear');
else
    power = NaN;
end

% Fallback only for low-end conditions
if isnan(speed) || isnan(power)
    if Q_des < Q_min       
        speed = speed_min / Q_min * Q_des;
         power = (speed / speed_min)^3 * P_min;

    else if h_des < h_min
        speed = speed_min * (h_des / h_min)^(1/2);
        power = (speed / speed_min)^3 * P_min;

    else
        speed = 0;
        power = 0;
    end


end

end

== matlab function ARC_DTm/PROS1_3/MATLAB Function2 ==
  data: cperm input; cbrine output; Qperm input; Qbrine input; Qfeed input; cfeed input
function cbrine = fcn(cperm, Qperm, Qbrine, Qfeed, cfeed)

Wtot = Qfeed * cfeed;
Wperm = cperm * Qperm;

%account for NaN
if Qbrine > 0
cbrine = (Wtot - Wperm)/Qbrine;
else
    cbrine = 0;
end

== matlab function ARC_DTm/PROS2_2/MATLAB Function1 ==
  data: W input; h input; dh output
function dh = hydDiameter(W,h)

dh = 2*h*W/(h+W);

== matlab function ARC_DTm/PROS1_3/Subsystem/MATLAB Function ==
  data: T input; Pfeed input; Pperm input; A input; B input; cfeed input; cperm_prev input; Jw_prev input; dh input; L input; u input; Jw output; cperm output; deltaPi_bar output; cmem output
function [Jw, cperm, deltaPi_bar,cmem] = ROBehavior(T, Pfeed, Pperm, A, B, cfeed, cperm_prev,Jw_prev, dh, L, u)
    
    cmem = ConP(cfeed, T, dh, L, u, Jw_prev);
    [pi_feed] = osmPres(T,cmem);
    [pi_perm] = osmPres(T,cperm_prev);
    
    deltaPi_bar = pi_feed - pi_perm;
    [Jw, cperm] = solutionDiffusion(T, Pfeed, Pperm, A, B, cmem, cperm_prev, pi_feed, pi_perm);
   
end

== matlab function ARC_DTm/PROS2_1_Pump/MATLAB Function1 ==
  data: Q_des input; speed output; h_des input; power output
function [speed, power] = query_pump(Q_des, h_des)
% QUERY_PUMP Find pump speed, power, and efficiency given flow and head
%MUST UPDATE the pump_data call
%
% Inputs:
%   Q_des     - Desired flow rate (gpm)
%   h_des     - Desired added head (ft)
%   pump_data - Struct for a single pump (e.g. pump.pump_A)
%
% Outputs:
%   speed      - Interpolated speed
%   power      - Interpolated power
%   total_eff  - Interpolated total efficiency (%)
%   totalPower - Power demand accounting for efficiency (power / total_eff / 100)

persistent pump_data Q_min h_min speed_min  P_min
if isempty(pump_data)
    loaded = coder.load('Pumps\LookupTables.mat');
    pump_data = loaded.pump.RO_IS_pump;
    Q_min = min(pump_data.Q_grid(:));
    h_min = min(pump_data.H_grid(:));

    speed_min = interp2(pump_data.Q_grid, pump_data.H_grid, pump_data.speed_grid, Q_min, h_min, 'linear');
    P_min = interp2(pump_data.H_grid_pwr, pump_data.S_grid_pwr, pump_data.power_grid, h_min, speed_min, 'linear');

end

%zero flow conditions not present in the existing dataset.
if Q_des <= .1 * Q_min
    speed = 0;
    power = 0;
    total_eff = 0;
    return
end

% Normal lookup
speed = interp2(pump_data.Q_grid, pump_data.H_grid, ...
    pump_data.speed_grid, Q_des, h_des, 'linear');

if ~isnan(speed)
    power = interp2(pump_data.H_grid_pwr, pump_data.S_grid_pwr, ...
        pump_data.power_grid, h_des, speed, 'linear');
else
    power = NaN;
end

% Fallback only for low-end conditions
if isnan(speed) || isnan(power)
    if Q_des < Q_min       
        speed = speed_min / Q_min * Q_des;
         power = (speed / speed_min)^3 * P_min;

    else if h_des < h_min
        speed = speed_min * (h_des / h_min)^(1/2);
        power = (speed / speed_min)^3 * P_min;

    else
        speed = 0;
        power = 0;
    end


end


end

== matlab function ARC_DTm/PROS2_3_Pump/MATLAB Function1 ==
  data: Q_des input; speed output; h_des input; power output
function [speed, power] = query_pump(Q_des, h_des)
% QUERY_PUMP Find pump speed, power, and efficiency given flow and head
%MUST UPDATE the pump_data call
%
% Inputs:
%   Q_des     - Desired flow rate (gpm)
%   h_des     - Desired added head (ft)
%   pump_data - Struct for a single pump (e.g. pump.pump_A)
%
% Outputs:
%   speed      - Interpolated speed
%   power      - Interpolated power
%   total_eff  - Interpolated total efficiency (%)
%   totalPower - Power demand accounting for efficiency (power / total_eff / 100)

persistent pump_data Q_min h_min speed_min  P_min
if isempty(pump_data)
    loaded = coder.load('Pumps\LookupTables.mat');
    pump_data = loaded.pump.RO_IS_pump;
    Q_min = min(pump_data.Q_grid(:));
    h_min = min(pump_data.H_grid(:));

    speed_min = interp2(pump_data.Q_grid, pump_data.H_grid, pump_data.speed_grid, Q_min, h_min, 'linear');
    P_min = interp2(pump_data.H_grid_pwr, pump_data.S_grid_pwr, pump_data.power_grid, h_min, speed_min, 'linear');

end

%zero flow conditions not present in the existing dataset.
if Q_des <= .1 * Q_min
    speed = 0;
    power = 0;
    total_eff = 0;
    return
end

% Normal lookup
speed = interp2(pump_data.Q_grid, pump_data.H_grid, ...
    pump_data.speed_grid, Q_des, h_des, 'linear');

if ~isnan(speed)
    power = interp2(pump_data.H_grid_pwr, pump_data.S_grid_pwr, ...
        pump_data.power_grid, h_des, speed, 'linear');
else
    power = NaN;
end

% Fallback only for low-end conditions
if isnan(speed) || isnan(power)
    if Q_des < Q_min       
        speed = speed_min / Q_min * Q_des;
         power = (speed / speed_min)^3 * P_min;

    else if h_des < h_min
        speed = speed_min * (h_des / h_min)^(1/2);
        power = (speed / speed_min)^3 * P_min;

    else
        speed = 0;
        power = 0;
    end


end


end

== matlab function ARC_DTm/PROS2_3/MATLAB Function1 ==
  data: W input; h input; dh output
function dh = hydDiameter(W,h)

dh = 2*h*W/(h+W);

== matlab function ARC_DTm/PROS2_3/MATLAB Function2 ==
  data: cperm input; cbrine output; Qperm input; Qbrine input; Qfeed input; cfeed input
function cbrine = fcn(cperm, Qperm, Qbrine, Qfeed, cfeed)

Wtot = Qfeed * cfeed;
Wperm = cperm * Qperm;

%account for NaN
if Qbrine > 0
cbrine = (Wtot - Wperm)/Qbrine;
else
    cbrine = 0;
end

== matlab function ARC_DTm/PROS1_4/MATLAB Function2 ==
  data: cperm input; cbrine output; Qperm input; Qbrine input; Qfeed input; cfeed input
function cbrine = fcn(cperm, Qperm, Qbrine, Qfeed, cfeed)

Wtot = Qfeed * cfeed;
Wperm = cperm * Qperm;

%account for NaN
if Qbrine > 0
cbrine = (Wtot - Wperm)/Qbrine;
else
    cbrine = 0;
end

== matlab function ARC_DTm/PROS1_2/MATLAB Function1 ==
  data: W input; h input; dh output
function dh = hydDiameter(W,h)

dh = 2*h*W/(h+W);

== matlab function ARC_DTm/PROS1_2/MATLAB Function2 ==
  data: cperm input; cbrine output; Qperm input; Qbrine input; Qfeed input; cfeed input
function cbrine = fcn(cperm, Qperm, Qbrine, Qfeed, cfeed)

Wtot = Qfeed * cfeed;
Wperm = cperm * Qperm;

%account for NaN
if Qbrine > 0
cbrine = (Wtot - Wperm)/Qbrine;
else
    cbrine = 0;
end

== matlab function ARC_DTm/PROS2_2/MATLAB Function2 ==
  data: cperm input; cbrine output; Qperm input; Qbrine input; Qfeed input; cfeed input
function cbrine = fcn(cperm, Qperm, Qbrine, Qfeed, cfeed)

Wtot = Qfeed * cfeed;
Wperm = cperm * Qperm;

%account for NaN
if Qbrine > 0
cbrine = (Wtot - Wperm)/Qbrine;
else
    cbrine = 0;
end

== matlab function ARC_DTm/PROS1_2/Subsystem/MATLAB Function ==
  data: T input; Pfeed input; Pperm input; A input; B input; cfeed input; cperm_prev input; Jw_prev input; dh input; L input; u input; Jw output; cperm output; deltaPi_bar output
function [Jw, cperm, deltaPi_bar] = ROBehavior(T, Pfeed, Pperm, A, B, cfeed, cperm_prev,Jw_prev, dh, L, u)
    
    cmem = ConP(cfeed, T, dh, L, u, Jw_prev);

    [pi_feed] = osmPres(T,cmem);
    [pi_perm] = osmPres(T,cperm_prev);
    
    deltaPi_bar = pi_feed - pi_perm;
    [Jw, cperm] = solutionDiffusion(T, Pfeed, Pperm, A, B, cmem, cperm_prev, pi_feed, pi_perm);
   
end

== matlab function ARC_DTm/PROS2_2/Subsystem/MATLAB Function ==
  data: T input; Pfeed input; Pperm input; A input; B input; cfeed input; cperm_prev input; Jw_prev input; dh input; L input; u input; Jw output; cperm output; deltaPi_bar output
function [Jw, cperm, deltaPi_bar] = ROBehavior(T, Pfeed, Pperm, A, B, cfeed, cperm_prev,Jw_prev, dh, L, u)
   
    cmem = ConP(cfeed, T, dh, L, u, Jw_prev);
    [pi_feed] = osmPres(T,cmem);
    [pi_perm] = osmPres(T,cperm_prev);
    
    deltaPi_bar = pi_feed - pi_perm;
    [Jw, cperm] = solutionDiffusion(T, Pfeed, Pperm, A, B, cmem, cperm_prev, pi_feed, pi_perm);
end

== matlab function ARC_DTm/PROS2_3/Subsystem/MATLAB Function ==
  data: T input; Pfeed input; Pperm input; A input; B input; cfeed input; cperm_prev input; Jw_prev input; dh input; L input; u input; Jw output; cperm output; deltaPi_bar output
function [Jw, cperm, deltaPi_bar] = ROBehavior(T, Pfeed, Pperm, A, B, cfeed, cperm_prev,Jw_prev, dh, L, u)
   
    cmem = ConP(cfeed, T, dh, L, u, Jw_prev);
    [pi_feed] = osmPres(T,cmem);
    [pi_perm] = osmPres(T,cperm_prev);
    
    deltaPi_bar = pi_feed - pi_perm;
    [Jw, cperm] = solutionDiffusion(T, Pfeed, Pperm, A, B, cmem, cperm_prev, pi_feed, pi_perm);
end

== matlab function ARC_DTm/PROS1_4/Subsystem/MATLAB Function ==
  data: T input; Pfeed input; Pperm input; A input; B input; cfeed input; cperm_prev input; Jw_prev input; dh input; L input; u input; Jw output; cperm output; deltaPi_bar output; cmem output
function [Jw, cperm, deltaPi_bar,cmem] = ROBehavior(T, Pfeed, Pperm, A, B, cfeed, cperm_prev,Jw_prev, dh, L, u)
    
    cmem = ConP(cfeed, T, dh, L, u, Jw_prev);
    [pi_feed] = osmPres(T,cmem);
    [pi_perm] = osmPres(T,cperm_prev);
    
    deltaPi_bar = pi_feed - pi_perm;
    [Jw, cperm] = solutionDiffusion(T, Pfeed, Pperm, A, B, cmem, cperm_prev, pi_feed, pi_perm);
   
end
